simulink model "force_control"  (R2020b)
settings: Solver=FixedStepAuto  StartTime=0.0  StopTime=10  FixedStep=Ts  RelTol=1e-3
undefined symbols (not defined in the file): dqi, fd, invMd, K, KD, KF, KI, KP, Md, myRobot, qi, xr
settings Model: Creator=simon  LastModifiedBy=SimoneCremasco
settings SolverCC: ZeroCrossControl=DisableAll

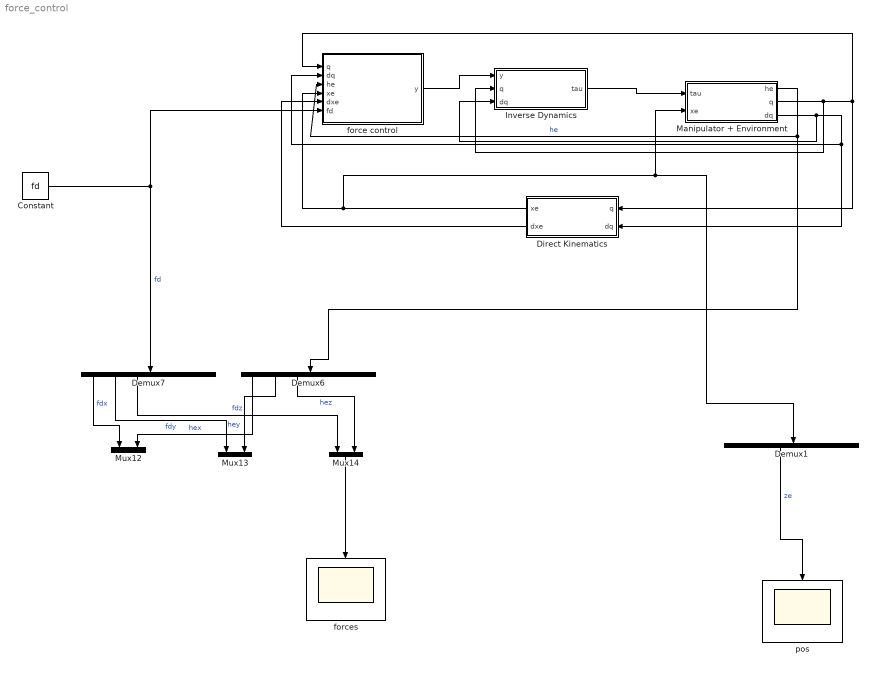
== system force_control ==
  Constant : Constant  Value=fd
  Demux1 : Demux  Outputs=6
  Demux6 : Demux  Outputs=6
  Demux7 : Demux  Outputs=6
  Direct Kinematics : Subsystem
  Inverse Dynamics : Subsystem
  Manipulator + Environment : Subsystem
  Mux12 : Mux  Inputs=2
  Mux13 : Mux  Inputs=2
  Mux14 : Mux  Inputs=2
  force control : Subsystem
  forces : Scope
  pos : Scope
  wires:
  Direct Kinematics/2(dxe) -> force control/5(dxe)
  force control/1(y) -> Inverse Dynamics/1(y)
  Inverse Dynamics/1(tau) -> Manipulator + Environment/1(tau)
  Manipulator + Environment/2(q) -> Inverse Dynamics/2(q), Direct Kinematics/1(q), force control/1(q)
  Manipulator + Environment/3(dq) -> Inverse Dynamics/3(dq), Direct Kinematics/2(dq), force control/2(dq)
  Manipulator + Environment/1(he) -> force control/3(he), Demux6/1  "he"
  Demux7/3 -> Mux14/1  "fdz"
  Direct Kinematics/1(xe) -> force control/4(xe), Demux1/1, Manipulator + Environment/2(xe)
  Constant/1 -> force control/6(fd), Demux7/1  "fd"
  Demux7/2 -> Mux13/1  "fdy"
  Demux7/1 -> Mux12/1  "fdx"
  Demux6/2 -> Mux13/2  "hey"
  Demux6/1 -> Mux12/2  "hex"
  Demux6/3 -> Mux14/2  "hez"
  Mux14/1 -> forces/1
  Demux1/3 -> pos/1  "ze"

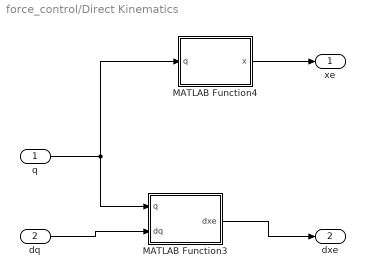
== system force_control/Direct Kinematics ==
  q : Inport
  dq : Inport  Port=2
  MATLAB Function3 : MATLAB Function  TreatAsAtomicUnit=on
  MATLAB Function4 : MATLAB Function  TreatAsAtomicUnit=on
  xe : Outport
  dxe : Outport  Port=2
  wires:
  MATLAB Function3/1(dxe) -> dxe/1
  dq/1 -> MATLAB Function3/2(dq)
  q/1 -> MATLAB Function4/1(q), MATLAB Function3/1(q)
  MATLAB Function4/1(x) -> xe/1

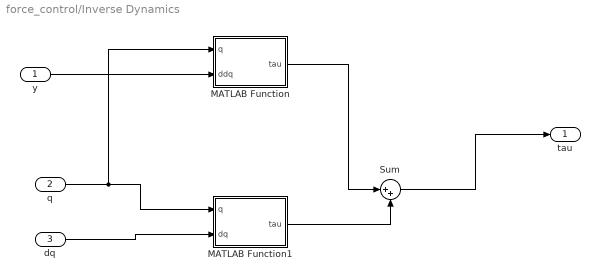
== system force_control/Inverse Dynamics ==
  y : Inport
  q : Inport  Port=2
  dq : Inport  Port=3
  MATLAB Function : MATLAB Function  TreatAsAtomicUnit=on
  MATLAB Function1 : MATLAB Function  TreatAsAtomicUnit=on
  Sum : Sum  Inputs=|++
  tau : Outport
  wires:
  MATLAB Function1/1(tau) -> Sum/2
  MATLAB Function/1(tau) -> Sum/1
  y/1 -> MATLAB Function/2(ddq)
  Sum/1 -> tau/1
  dq/1 -> MATLAB Function1/2(dq)
  q/1 -> MATLAB Function/1(q), MATLAB Function1/1(q)

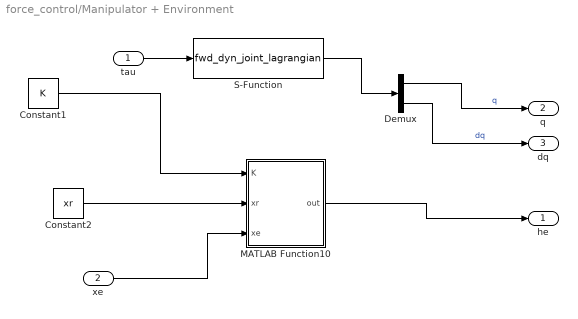
== system force_control/Manipulator + Environment ==
  tau : Inport
  xe : Inport  Port=2
  Constant1 : Constant  Value=K
  Constant2 : Constant  Value=xr
  Demux : Demux  Outputs=2
  MATLAB Function10 : MATLAB Function  TreatAsAtomicUnit=on
  S-Function : S-Function  FunctionName=fwd_dyn_joint_lagrangian  Parameters=myRobot,qi,dqi  SFunctionDeploymentMode=off  EnableBusSupport=off
  he : Outport
  q : Outport  Port=2
  dq : Outport  Port=3
  wires:
  tau/1 -> S-Function/1
  Constant1/1 -> MATLAB Function10/1(K)
  Constant2/1 -> MATLAB Function10/2(xr)
  xe/1 -> MATLAB Function10/3(xe)
  S-Function/1 -> Demux/1
  Demux/1 -> q/1  "q"
  Demux/2 -> dq/1  "dq"
  MATLAB Function10/1(out) -> he/1

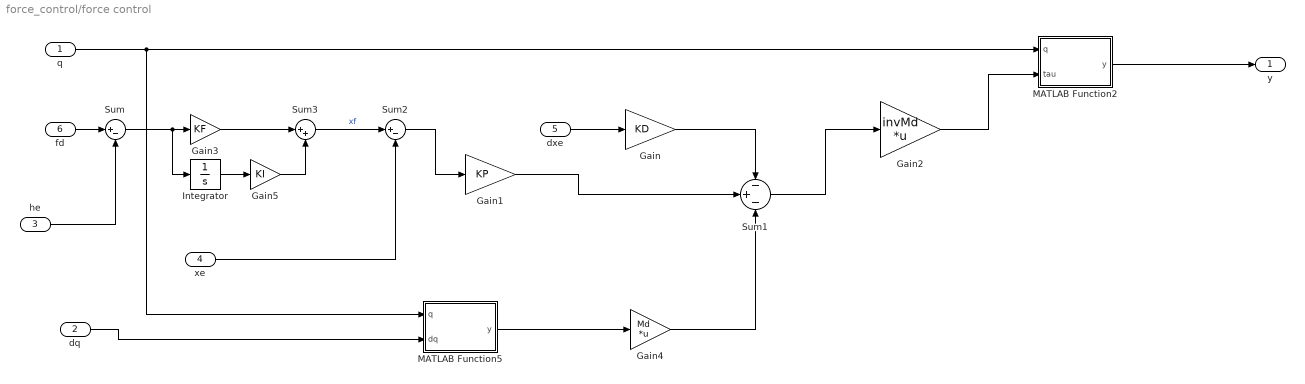
== system force_control/force control ==
  q : Inport
  dq : Inport  Port=2
  he : Inport  Port=3
  xe : Inport  Port=4
  dxe : Inport  Port=5
  fd : Inport  Port=6
  Gain : Gain  Gain=KD
  Gain1 : Gain  Gain=KP
  Gain2 : Gain  Gain=invMd  Multiplication=Matrix(K*u)
  Gain3 : Gain  Gain=KF
  Gain4 : Gain  Gain=Md  Multiplication=Matrix(K*u)
  Gain5 : Gain  Gain=KI
  Integrator : Integrator
  MATLAB Function2 : MATLAB Function  TreatAsAtomicUnit=on
  MATLAB Function5 : MATLAB Function  TreatAsAtomicUnit=on
  Sum : Sum  Inputs=|+-
  Sum1 : Sum  Inputs=-+-
  Sum2 : Sum  Inputs=|+-
  Sum3 : Sum  Inputs=|++
  y : Outport
  wires:
  MATLAB Function5/1(y) -> Gain4/1
  Gain2/1 -> MATLAB Function2/2(tau)
  MATLAB Function2/1(y) -> y/1
  dxe/1 -> Gain/1
  Sum1/1 -> Gain2/1
  Sum2/1 -> Gain1/1
  q/1 -> MATLAB Function5/1(q), MATLAB Function2/1(q)
  dq/1 -> MATLAB Function5/2(dq)
  Gain/1 -> Sum1/1
  xe/1 -> Sum2/2
  Gain1/1 -> Sum1/2
  Gain4/1 -> Sum1/3
  fd/1 -> Sum/1
  Sum/1 -> Integrator/1, Gain3/1
  he/1 -> Sum/2
  Integrator/1 -> Gain5/1
  Gain3/1 -> Sum3/1
  Gain5/1 -> Sum3/2
  Sum3/1 -> Sum2/1  "xf"

== matlab function force_control/force control/MATLAB Function5 ==
  data: q input; y output; dq input
function y = dJa(q, dq)

y = getDiffJa(q)*dq;

== matlab function force_control/Direct Kinematics/MATLAB Function3 ==
  data: q input; dxe output; dq input
function dxe = Ja(q, dq)

dxe = getJa(q)*dq;

== matlab function force_control/force control/MATLAB Function2 ==
  data: q input; y output; tau input
function y = invJa(q, tau)

y = getInvJa(q)*tau;

== matlab function force_control/Direct Kinematics/MATLAB Function4 ==
  data: q input; x output
function x = k(q)

x = getK(q);

== matlab function force_control/Inverse Dynamics/MATLAB Function ==
  data: q input size=3; tau output; ddq input size=3
function tau = B(q, ddq)

tau = getB(q)*ddq;

== matlab function force_control/Inverse Dynamics/MATLAB Function1 ==
  data: q input size=3; tau output; dq input size=3
function tau = n(q, dq)

tau = getN(q, dq);

== matlab function force_control/Manipulator + Environment/MATLAB Function10 ==
  data: K input; out output size=6; xr input; xe input size=6
function out = hde(K,xr, xe)
%consider the interaction only in z direction
if xe(3) < xr(3)
    out = K*(xe-xr);
else 
    out = zeros(6,1);
end
